simulink model "exnb4137986_Q5"  (R2024b)
settings: Solver=FixedStepAuto  StartTime=0.0  StopTime=5  FixedStep=0.001  RelTol=1e-3
values from neighbouring files (symbols this model uses):
  u_star_1 = double(u_star_1)    [exnb4137986_Q10_par.m]    (also in exnb4137986_Q4_par.m = double(subs(u_eq, ss_states, x_star_1)); exnb4137986_Q5_par.m; exnb4137986_Q7_par.m; exnb4137986_Q8_par.m)
  values = [0, 0.01, 1, 0.001, 1, 1, 10]    [exnb4137986_Q10_par.m]    (also in exnb4137986_Q4_par.m; exnb4137986_Q5_par.m; exnb4137986_Q7_par.m; exnb4137986_Q8_par.m)
  x_star_1 = [I_star_1, omega_star_1]    [exnb4137986_Q10_par.m]    (also in exnb4137986_Q4_par.m = [omega_star_1, I_star_1]; exnb4137986_Q5_par.m; exnb4137986_Q7_par.m; exnb4137986_Q8_par.m)
settings Model: Creator=therkelsen  LastModifiedBy=therkelsen

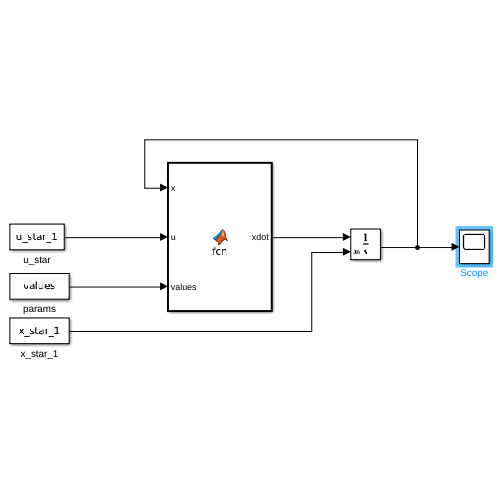
[thumbnail: Simulink's stored preview of the top-level diagram]
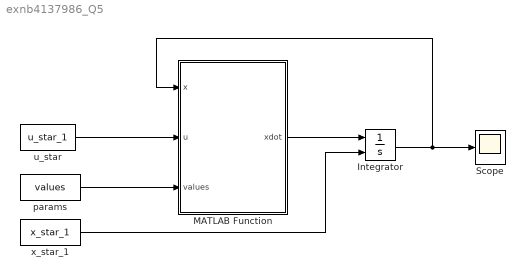
== system exnb4137986_Q5 ==
  Integrator : Integrator  InitialConditionSource=external
  MATLAB Function : MATLAB Function  TreatAsAtomicUnit=on
  Scope : Scope
  params : Constant  Value=values
  u_star : Constant  Value=u_star_1
  x_star_1 : Constant  Value=x_star_1
  wires:
  x_star_1/1 -> Integrator/2
  Integrator/1 -> Scope/1, MATLAB Function/1(x)
  MATLAB Function/1(xdot) -> Integrator/1
  params/1 -> MATLAB Function/3(values)
  u_star/1 -> MATLAB Function/2(u)

== matlab function exnb4137986_Q5/MATLAB Function ==
  data: x input; u input; xdot output; values input
function xdot = fcn(x, u, values)

J = values(2);
L = values(3);
Kd = values(4);
Ke = values(5);
Km = values(6);
Rm = values(7);

xdot = [-Rm/L * x(1) - Ke/L * x(2) + 1/L * u;
         Km/J * x(1) - Kd/J * x(2)];
